simulink model "s10_10"  (Simulink 6.6)
settings: Solver=ode45  SolverMode=SingleTasking  StartTime=0.0  StopTime=t_d  MaxStep=Tc  RelTol=1e-6  AbsTol=1e-6
values from neighbouring files (symbols this model uses):
  g = 9.81    [i10_10.m]
  K_d = diag([330; 330; 165; 40])    [i10_10.m]
  K_p = diag([300; 300; 150; 50])    [i10_10.m]
  m3 = 2    [i10_10.m]
  pi_l = pi_m    [i10_10.m]
  q_i = inv_ksu(a,x_i)    [i10_10.m]
  Tc = 0.04    [i10_10.m]
  Ts = Tc    (= 0.04)    [i10_10.m]
  x_do = [-0.1; 0.1; 0.6; -pi/3]    [i10_10.m]
  x_o = [1; 1; 1; pi/4]    [i10_10.m]
undefined symbols (not defined in the file or in its folder): a, iner_s
settings Model: Creator=luigivillani  LastModifiedBy=luigivillani  ExtModeAutoUpdateStatusClock=off
settings DataIOCC: LimitDataPoints=off  SaveOutput=off  SaveTime=off  SignalLoggingName=sigsOut
settings OptimizationCC: BooleanDataType=off
settings DebuggingCC: SignalResolutionControl=TryResolveAllWithWarning  SolverPrmCheckMsg=none  MultiTaskDSMMsg=warning  MultiTaskCondExecSysMsg=none  StrictBusMsg=None
settings HardwareCC: TargetUnknown=on
settings RTWCC: IncludeERTFirstTime=on

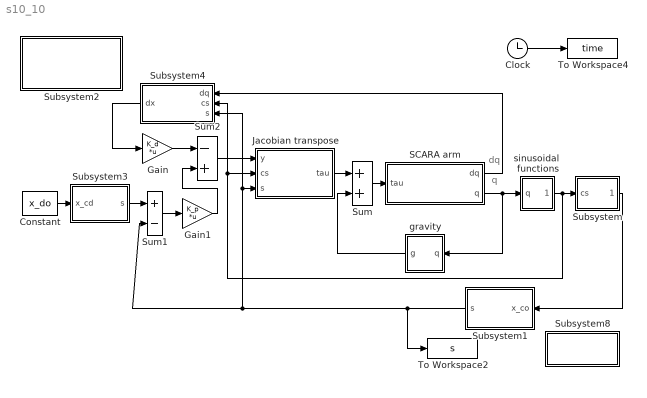
== system s10_10 ==
  note: dq
  note: q
  Clock : Clock
      settings: Decimation=10
  Constant : Constant  Value=x_do  SampleTime=Tc
  Gain : Gain  Gain=K_d  Multiplication=Matrix(K*u)  SampleTime=Tc
      mask Display: disp('K_d')
  Gain1 : Gain  Gain=K_p  Multiplication=Matrix(K*u)  SampleTime=Tc
      mask Display: disp('K_p')
  Jacobian transpose : Subsystem
      mask Display: disp('tr(J_L(s,zc,q))')
  SCARA arm : Subsystem
      mask Display: disp('inv(B(q))(tau-tau'')')
  Subsystem : Subsystem
  Subsystem1 : Subsystem  Orientation=left
      mask Display: disp('features')
  Subsystem2 : Subsystem
      settings: OpenFcn=clear all;i10_10;
      mask Display: disp('variables\n initialization')
  Subsystem3 : Subsystem
      mask Display: disp('features')
  Subsystem4 : Subsystem  Orientation=left
      mask Display: disp('J_L(s,zc,q)')
  Subsystem8 : Subsystem
      settings: OpenFcn=p10_10;
      mask Display: disp('plot')
  Sum : Sum  SaturateOnIntegerOverflow=on  InputSameDT=on
  Sum1 : Sum  Inputs=+-  SaturateOnIntegerOverflow=on  InputSameDT=on
  Sum2 : Sum  Inputs=-+  SaturateOnIntegerOverflow=on  InputSameDT=on
  To Workspace2 : ToWorkspace  VariableName=s  SampleTime=Ts  SaveFormat=Array
      settings: MaxDataPoints=4001
  To Workspace4 : ToWorkspace  VariableName=time  SampleTime=Ts  SaveFormat=Array
      settings: MaxDataPoints=4001
  gravity : Subsystem  Orientation=left
      mask Display: disp('g(q)')
  sinusoidal  functions : Subsystem
      mask Display: disp('cs(q)')
  wires:
  Sum/1 -> SCARA arm/1(tau)
  Clock/1 -> To Workspace4/1
  Constant/1 -> Subsystem3/1(x_cd)
  gravity/1(g) -> Sum/2
  Jacobian transpose/1(tau) -> Sum/1
  SCARA arm/2("q ") -> sinusoidal  functions/1(q), gravity/1(q)
  Sum2/1 -> Jacobian transpose/1(y)
  Gain/1 -> Sum2/1
  Subsystem4/1(dx) -> Gain/1
  SCARA arm/1(dq) -> Subsystem4/1(dq)
  Gain1/1 -> Sum2/2
  Sum1/1 -> Gain1/1
  sinusoidal  functions/1(cs) -> Subsystem/1(cs), Jacobian transpose/2(cs), Subsystem4/2(cs)
  Subsystem1/1(s) -> To Workspace2/1, Sum1/2, Subsystem4/3(s), Jacobian transpose/3(s)
  Subsystem/1(x_co) -> Subsystem1/1(x_co)
  Subsystem3/1(s) -> Sum1/1

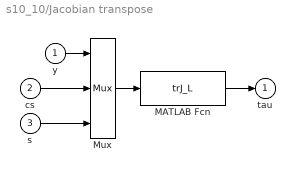
== system s10_10/Jacobian transpose ==
  y : Inport
  cs : Inport  Port=2
  s : Inport  Port=3
  MATLAB Fcn : MATLABFcn  MATLABFcn=trJ_L  OutputDimensions=4  SampleTime=Tc
      mask Display: disp('J''_L(s,zc,q)y')
  Mux : Mux  Inputs=[4,6,4]
  tau : Outport  InitialOutput=0
  wires:
  MATLAB Fcn/1 -> tau/1
  Mux/1 -> MATLAB Fcn/1
  cs/1 -> Mux/2
  y/1 -> Mux/1
  s/1 -> Mux/3

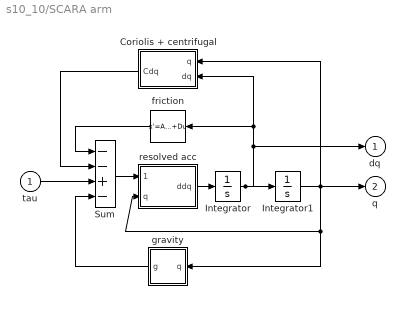
== system s10_10/SCARA arm ==
  tau : Inport
  Coriolis + centrifugal : Subsystem  Orientation=left
      mask Display: disp('C(q,dq)dq')
  Integrator : Integrator  InitialCondition=[0 0 0 0]
  Integrator1 : Integrator  InitialCondition=q_i
  Sum : Sum  Inputs=--+-  SaturateOnIntegerOverflow=on  InputSameDT=on
  friction : StateSpace  Orientation=left  A=[]  B=[]  C=[]  D=K  mask(Matrix Gain){@1=F_v}
      mask prompts: @1 "Gain matrix:"
      mask help: Matrix Gain.
      mask init:
      | K = @1;
      mask Help: Multiplies input vector by entered matrix to produce output vector (y=Au).
      mask Display: disp('F_v')
  gravity : Subsystem  Orientation=left
      mask Display: disp('g(q)')
  resolved acc : Subsystem
      mask Display: disp('inv(B(q))')
  dq : Outport  InitialOutput=0
  "q " : Outport  Port=2  InitialOutput=0
  wires:
  Coriolis + centrifugal/1(Cdq) -> Sum/2
  tau/1 -> Sum/3
  Integrator1/1 -> Coriolis + centrifugal/1(q), resolved acc/2(q), gravity/1(q), "q "/1
  resolved acc/1(ddq) -> Integrator/1
  Integrator/1 -> Integrator1/1, dq/1, friction/1, Coriolis + centrifugal/2(dq)
  Sum/1 -> resolved acc/1(tau-tau')
  friction/1 -> Sum/1
  gravity/1(g) -> Sum/4

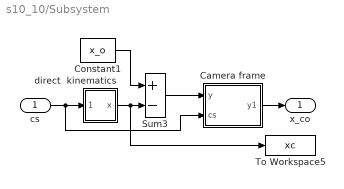
== system s10_10/Subsystem ==
  cs : Inport
  Camera frame : Subsystem
      mask Display: disp('c_frame')
  Constant1 : Constant  Value=x_o  SampleTime=Tc
  Sum3 : Sum  Inputs=+-  SaturateOnIntegerOverflow=on  InputSameDT=on
  To Workspace5 : ToWorkspace  VariableName=xc  SampleTime=Ts  SaveFormat=Array
      settings: MaxDataPoints=4001
  direct  kinematics : Subsystem
      mask Display: disp('k(q)')
  x_co : Outport
  wires:
  Constant1/1 -> Sum3/1
  direct  kinematics/1(x) -> To Workspace5/1, Sum3/2
  Sum3/1 -> Camera frame/1(y)
  cs/1 -> direct  kinematics/1(cs), Camera frame/2(cs)
  Camera frame/1(y1) -> x_co/1

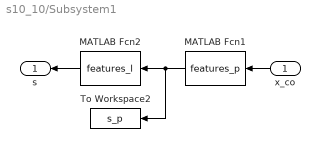
== system s10_10/Subsystem1 ==
  x_co : Inport  Orientation=left
  MATLAB Fcn1 : MATLABFcn  Orientation=left  MATLABFcn=features_p  OutputDimensions=4  SampleTime=Tc
      mask Display: disp('points')
  MATLAB Fcn2 : MATLABFcn  Orientation=left  MATLABFcn=features_l  OutputDimensions=4
      mask Display: disp('line')
  To Workspace2 : ToWorkspace  VariableName=s_p  SampleTime=Ts  SaveFormat=Array
      settings: MaxDataPoints=4001
  s : Outport  Orientation=left
  wires:
  MATLAB Fcn1/1 -> MATLAB Fcn2/1, To Workspace2/1
  x_co/1 -> MATLAB Fcn1/1
  MATLAB Fcn2/1 -> s/1

== system s10_10/Subsystem2 ==
  note: start

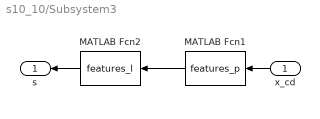
== system s10_10/Subsystem3 ==
  x_cd : Inport  Orientation=left
  MATLAB Fcn1 : MATLABFcn  Orientation=left  MATLABFcn=features_p  OutputDimensions=4  SampleTime=Tc
      mask Display: disp('points')
  MATLAB Fcn2 : MATLABFcn  Orientation=left  MATLABFcn=features_l  OutputDimensions=4
      mask Display: disp('line')
  s : Outport  Orientation=left
  wires:
  MATLAB Fcn1/1 -> MATLAB Fcn2/1
  x_cd/1 -> MATLAB Fcn1/1
  MATLAB Fcn2/1 -> s/1

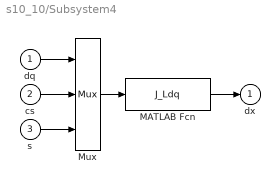
== system s10_10/Subsystem4 ==
  dq : Inport
  cs : Inport  Port=2
  s : Inport  Port=3
  MATLAB Fcn : MATLABFcn  MATLABFcn=J_Ldq  OutputDimensions=4  SampleTime=Tc
      mask Display: disp('J_L(s,zc,q)dq')
  Mux : Mux  Inputs=[4,6,4]
  dx : Outport  InitialOutput=0
  wires:
  dq/1 -> Mux/1
  cs/1 -> Mux/2
  Mux/1 -> MATLAB Fcn/1
  MATLAB Fcn/1 -> dx/1
  s/1 -> Mux/3

== system s10_10/Subsystem8 ==
  note: start

== system s10_10/gravity ==
  q : Inport  Orientation=left
  Constant : Constant  Orientation=left  Value=[0;0;m3*g;0]  SampleTime=Tc
  Terminator : Terminator
  g : Outport  Orientation=left  InitialOutput=0
  wires:
  q/1 -> Terminator/1
  Constant/1 -> g/1

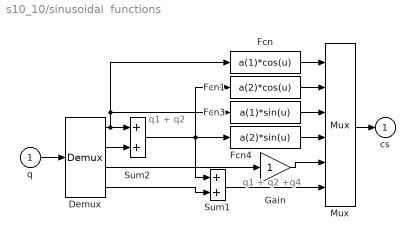
== system s10_10/sinusoidal  functions ==
  note: q1 + q2
  note: q1 + q2 +q4
  q : Inport
  Demux : Demux
  Fcn : Fcn  Expr=a(1)*cos(u)  SampleTime=Tc
  Fcn1 : Fcn  Expr=a(2)*cos(u)  SampleTime=Tc
  Fcn3 : Fcn  Expr=a(1)*sin(u)  SampleTime=Tc
  Fcn4 : Fcn  Expr=a(2)*sin(u)  SampleTime=Tc
  Gain : Gain  SampleTime=Tc
  Mux : Mux  Inputs=6
  Sum1 : Sum  SampleTime=Tc  SaturateOnIntegerOverflow=on  InputSameDT=on
  Sum2 : Sum  SampleTime=Tc  SaturateOnIntegerOverflow=on  InputSameDT=on
  cs : Outport  InitialOutput=0
  wires:
  Fcn/1 -> Mux/1
  Mux/1 -> cs/1
  Demux/2 -> Sum2/2
  Sum2/1 -> Fcn1/1, Fcn4/1, Sum1/1
  Demux/1 -> Sum2/1, Fcn/1, Fcn3/1
  Fcn1/1 -> Mux/2
  Fcn3/1 -> Mux/3
  Fcn4/1 -> Mux/4
  q/1 -> Demux/1
  Demux/4 -> Sum1/2
  Sum1/1 -> Mux/6
  Demux/3 -> Gain/1
  Gain/1 -> Mux/5

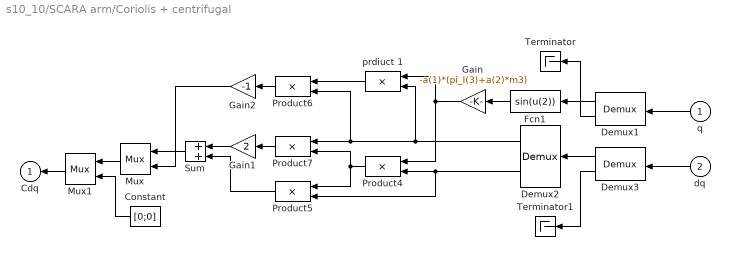
== system s10_10/SCARA arm/Coriolis + centrifugal ==
  q : Inport  Orientation=left
  dq : Inport  Orientation=left  Port=2
  Constant : Constant  Orientation=left  Value=[0;0]
  Demux1 : Demux  Orientation=left  Outputs=2
  Demux2 : Demux  Orientation=left  Outputs=2
  Demux3 : Demux  Orientation=left  Outputs=2
  Fcn1 : Fcn  Orientation=left  Expr=sin(u(2))
  Gain : Gain  Orientation=left  Gain=-a(1)*(pi_l(3)+a(2)*m3)  SaturateOnIntegerOverflow=on
      mask Display: disp('k_3')
  Gain1 : Gain  Orientation=left  Gain=2  SaturateOnIntegerOverflow=on
  Gain2 : Gain  Orientation=left  Gain=-1  SaturateOnIntegerOverflow=on
  Mux : Mux  Orientation=left  Inputs=2
  Mux1 : Mux  Orientation=left  Inputs=[2 2]
  Product{4..7} (4 alike) : Product  Orientation=left  SaturateOnIntegerOverflow=on  InputSameDT=on
  Sum : Sum  Orientation=left  SaturateOnIntegerOverflow=on  InputSameDT=on
  Terminator : Terminator
  Terminator1 : Terminator
  prdiuct 1 : Product  Orientation=left  SaturateOnIntegerOverflow=on  InputSameDT=on
  Cdq : Outport  Orientation=left  InitialOutput=0
  wires:
  Gain2/1 -> Mux/2
  Product6/1 -> Gain2/1
  Sum/1 -> Mux/1
  Product5/1 -> Sum/2
  Gain1/1 -> Sum/1
  Product7/1 -> Gain1/1
  Demux2/1 -> prdiuct 1/2, Product6/2, Product7/1
  Demux2/2 -> Product4/2, Product5/2
  prdiuct 1/1 -> Product6/1
  Gain/1 -> prdiuct 1/1, Product4/1
  Fcn1/1 -> Gain/1
  Product4/1 -> Product5/1, Product7/2
  q/1 -> Demux1/1
  dq/1 -> Demux3/1
  Demux1/1 -> Fcn1/1
  Demux3/1 -> Demux2/1
  Mux1/1 -> Cdq/1
  Mux/1 -> Mux1/1
  Constant/1 -> Mux1/2
  Demux1/2 -> Terminator/1
  Demux3/2 -> Terminator1/1

== system s10_10/SCARA arm/gravity ==
  q : Inport  Orientation=left
  Constant : Constant  Orientation=left  Value=[0;0; m3*g;0]
  Terminator : Terminator
  g : Outport  Orientation=left  InitialOutput=0
  wires:
  q/1 -> Terminator/1
  Constant/1 -> g/1

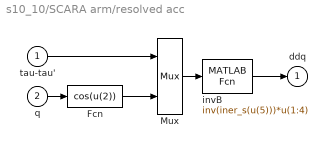
== system s10_10/SCARA arm/resolved acc ==
  tau-tau' : Inport
  q : Inport  Port=2
  Fcn : Fcn  Expr=cos(u(2))
  Mux : Mux  Inputs=[4,1]
  "invB " : MATLABFcn  MATLABFcn=inv(iner_s(u(5)))*u(1:4)  OutputDimensions=4
      mask Display: disp('inv(B(q))')
  ddq : Outport  InitialOutput=0
  wires:
  Fcn/1 -> Mux/2
  q/1 -> Fcn/1
  tau-tau'/1 -> Mux/1
  Mux/1 -> "invB "/1
  "invB "/1 -> ddq/1

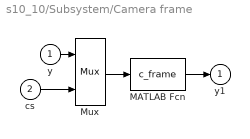
== system s10_10/Subsystem/Camera frame ==
  y : Inport
  cs : Inport  Port=2
  MATLAB Fcn : MATLABFcn  MATLABFcn=c_frame  OutputDimensions=4
      mask Display: disp('c_frame')
  Mux : Mux  Inputs=[4,6]
  y1 : Outport  InitialOutput=0
  wires:
  MATLAB Fcn/1 -> y1/1
  Mux/1 -> MATLAB Fcn/1
  y/1 -> Mux/1
  cs/1 -> Mux/2

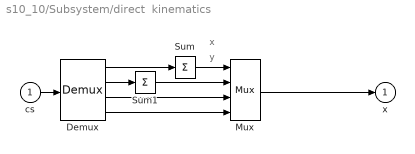
== system s10_10/Subsystem/direct  kinematics ==
  note: y
  note: x
  cs : Inport
  Demux : Demux  Outputs=[2,2,1,1]
  Mux : Mux
  Sum : Sum  Inputs=+  SaturateOnIntegerOverflow=on  InputSameDT=on
  Sum1 : Sum  Inputs=+  SaturateOnIntegerOverflow=on  InputSameDT=on
  x : Outport  InitialOutput=0
  wires:
  Sum1/1 -> Mux/2
  Sum/1 -> Mux/1
  Demux/2 -> Sum1/1
  Demux/1 -> Sum/1
  cs/1 -> Demux/1
  Mux/1 -> x/1
  Demux/4 -> Mux/4
  Demux/3 -> Mux/3
